simulink model "project"  (R2024a)
settings: Solver=VariableStepAuto  StartTime=0.0  StopTime=10.0  RelTol=1e-3
settings Model: Creator=DELL  LastModifiedBy=DELL

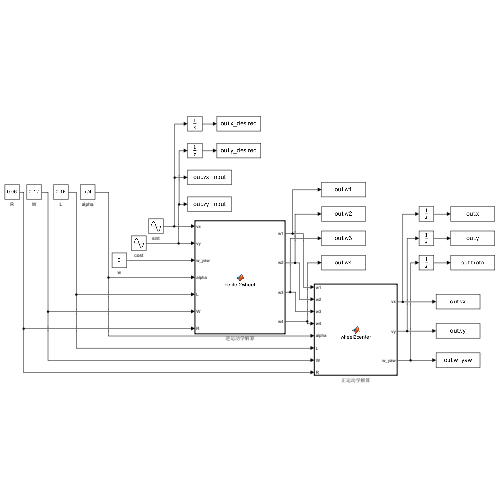
[thumbnail: Simulink's stored preview of the top-level diagram]
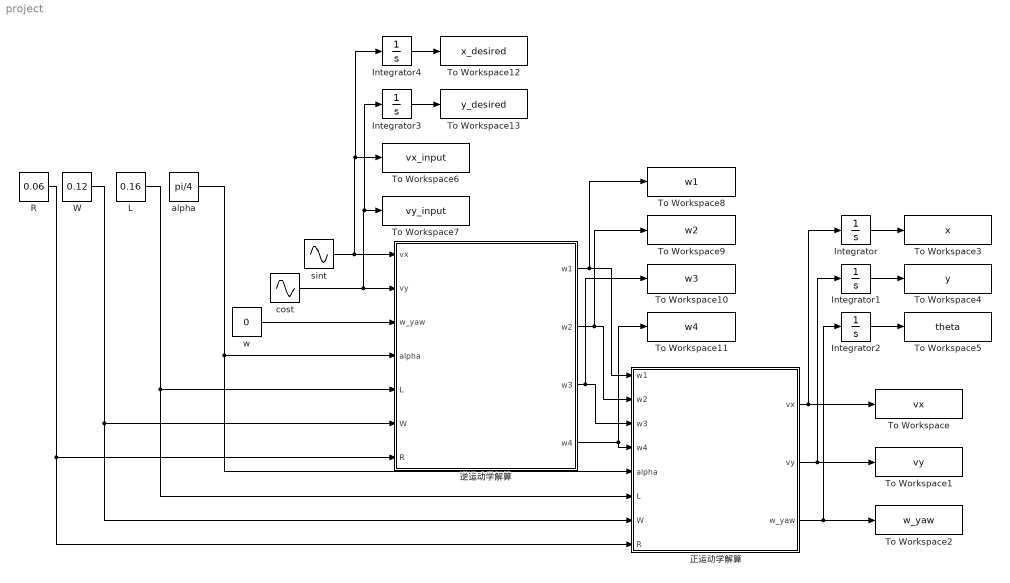
== system project ==
  Integrator{,1..4} (5 alike) : Integrator
  L : Constant  Value=0.16
  R : Constant  Value=0.06
  To Workspace : ToWorkspace  VariableName=vx  SaveFormat=Timeseries  SampleTime=-1
  To Workspace1 : ToWorkspace  VariableName=vy  SaveFormat=Timeseries  SampleTime=-1
  To Workspace10 : ToWorkspace  VariableName=w3  SaveFormat=Timeseries  SampleTime=-1
  To Workspace11 : ToWorkspace  VariableName=w4  SaveFormat=Timeseries  SampleTime=-1
  To Workspace12 : ToWorkspace  VariableName=x_desired  SaveFormat=Timeseries  SampleTime=-1
  To Workspace13 : ToWorkspace  VariableName=y_desired  SaveFormat=Timeseries  SampleTime=-1
  To Workspace2 : ToWorkspace  VariableName=w_yaw  SaveFormat=Timeseries  SampleTime=-1
  To Workspace3 : ToWorkspace  VariableName=x  SaveFormat=Timeseries  SampleTime=-1
  To Workspace4 : ToWorkspace  VariableName=y  SaveFormat=Timeseries  SampleTime=-1
  To Workspace5 : ToWorkspace  VariableName=theta  SaveFormat=Timeseries  SampleTime=-1
  To Workspace6 : ToWorkspace  VariableName=vx_input  SaveFormat=Timeseries  SampleTime=-1
  To Workspace7 : ToWorkspace  VariableName=vy_input  SaveFormat=Timeseries  SampleTime=-1
  To Workspace8 : ToWorkspace  VariableName=w1  SaveFormat=Timeseries  SampleTime=-1
  To Workspace9 : ToWorkspace  VariableName=w2  SaveFormat=Timeseries  SampleTime=-1
  W : Constant  Value=0.12
  alpha : Constant  Value=pi/4
  cost : Sin  Phase=pi/2  SampleTime=0
  sint : Sin  SampleTime=0
  w : Constant  Value=0
  正运动学解算 : MATLAB Function  TreatAsAtomicUnit=on
  逆运动学解算 : MATLAB Function  TreatAsAtomicUnit=on
  wires:
  alpha/1 -> 正运动学解算/5(alpha), 逆运动学解算/4(alpha)
  L/1 -> 正运动学解算/6(L), 逆运动学解算/5(L)
  W/1 -> 正运动学解算/7(W), 逆运动学解算/6(W)
  R/1 -> 正运动学解算/8(R), 逆运动学解算/7(R)
  w/1 -> 逆运动学解算/3(w_yaw)
  cost/1 -> Integrator3/1, To Workspace7/1, 逆运动学解算/2(vy)
  sint/1 -> Integrator4/1, To Workspace6/1, 逆运动学解算/1(vx)
  逆运动学解算/1(w1) -> To Workspace8/1, 正运动学解算/1(w1)
  逆运动学解算/2(w2) -> To Workspace9/1, 正运动学解算/2(w2)
  逆运动学解算/3(w3) -> To Workspace10/1, 正运动学解算/3(w3)
  逆运动学解算/4(w4) -> To Workspace11/1, 正运动学解算/4(w4)
  正运动学解算/1(vx) -> To Workspace/1, Integrator/1
  正运动学解算/2(vy) -> To Workspace1/1, Integrator1/1
  正运动学解算/3(w_yaw) -> Integrator2/1, To Workspace2/1
  Integrator/1 -> To Workspace3/1
  Integrator1/1 -> To Workspace4/1
  Integrator2/1 -> To Workspace5/1
  Integrator4/1 -> To Workspace12/1
  Integrator3/1 -> To Workspace13/1

== matlab function project/逆运动学解算 ==
  data: vx input; w1 output; vy input; w_yaw input; alpha input; L input; W input; R input; w2 output; w3 output; w4 output
function [w1,w2,w3,w4] = center2wheel(vx,vy,w_yaw,alpha,L,W,R)
%args:
% vx：整车x方向速度分量
% vy：整车y方向速度分量
% w_yaw：整车绕yaw轴角速度，逆时针为正
% alpha:接触地面的辊子的轴线与麦克纳姆轮轴线的夹角
% L：小车底盘左右轮轮心距的一半
% W：小车底盘前后轮轮心距的一半
% R：轮子半径

%return:
%w1:右上
%w2:左上
%w3:左下
%w4:右下
offset = w_yaw * (L + W * cot(alpha));

w1 = (-vx * cot(alpha) + vy + offset)/R;
w2 = (vx * cot(alpha) + vy - offset)/R;
w3 = (-vx * cot(alpha) + vy - offset)/R;
w4 = (vx * cot(alpha) + vy + offset)/R;

end

== matlab function project/正运动学解算 ==
  data: w1 input; vx output; w2 input; w3 input; w4 input; alpha input; L input; W input; R input; vy output; w_yaw output
function [vx,vy,w_yaw] = wheel2center(w1,w2,w3,w4,alpha,L,W,R)
arg = 4*cot(alpha);

%底盘输出速度
vx = -(R*(w1 - w2 + w3 - w4))/arg;
vy = (R*(w1 + w2 + w3 + w4))/4;
w_yaw = (R*(w1 - w2 - w3 + w4))/(4*L + W*arg);

end
